simulink model "Punto_3"  (R2020a)
settings: Solver=VariableStepAuto  StartTime=0.0  StopTime=10.0  RelTol=1e-3
undefined symbols (not defined in the file): t0
libraries: simulink x3
settings Model: Creator=nicoquintero  LastModifiedBy=nicoquintero

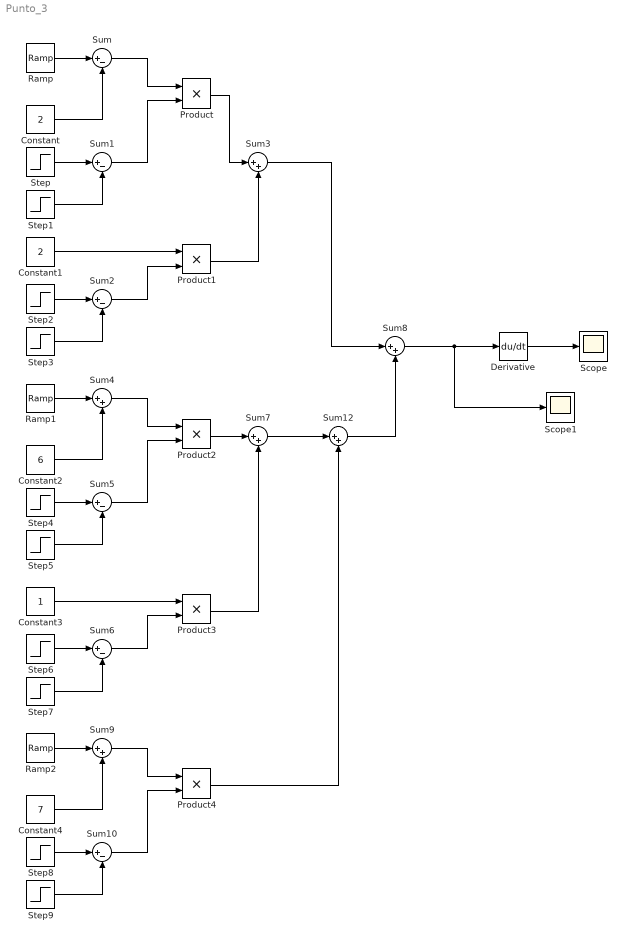
== system Punto_3 ==
  Constant : Constant  Value=2
  Constant1 : Constant  Value=2
  Constant2 : Constant  Value=6
  Constant3 : Constant
  Constant4 : Constant  Value=7
  Derivative : Derivative
  Product{,1..4} (5 alike) : Product
  Ramp : simulink/Sources/Ramp  slope=2  start=t0  InitialOutput=0
  Ramp1 : simulink/Sources/Ramp  slope=-1  start=t0  InitialOutput=0
  Ramp2 : simulink/Sources/Ramp  slope=-1  start=t0  InitialOutput=0
  Scope : Scope
  Scope1 : Scope
  Step : Step  Time=t0  SampleTime=0
  Step1 : Step  Time=t0+2  SampleTime=0
  Step2 : Step  Time=t0+2  SampleTime=0
  Step3 : Step  Time=t0+3  SampleTime=0
  Step4 : Step  Time=t0+3  SampleTime=0
  Step5 : Step  Time=t0+5  SampleTime=0
  Step6 : Step  Time=t0+5  SampleTime=0
  Step7 : Step  Time=t0+6  SampleTime=0
  Step8 : Step  Time=t0+6  SampleTime=0
  Step9 : Step  Time=t0+8  SampleTime=0
  Sum{,1..2,5..6,10} (6 alike) : Sum  Inputs=|+-
  Sum{3..4,7..9,12} (6 alike) : Sum  Inputs=|++
  wires:
  Ramp/1 -> Sum/1
  Constant/1 -> Sum/2
  Step/1 -> Sum1/1
  Step1/1 -> Sum1/2
  Sum1/1 -> Product/2
  Sum/1 -> Product/1
  Step2/1 -> Sum2/1
  Step3/1 -> Sum2/2
  Constant1/1 -> Product1/1
  Sum2/1 -> Product1/2
  Product1/1 -> Sum3/2
  Product/1 -> Sum3/1
  Step5/1 -> Sum5/2
  Sum5/1 -> Product2/2
  Step4/1 -> Sum5/1
  Constant2/1 -> Sum4/2
  Sum4/1 -> Product2/1
  Ramp1/1 -> Sum4/1
  Step7/1 -> Sum6/2
  Constant3/1 -> Product3/1
  Product3/1 -> Sum7/2
  Sum6/1 -> Product3/2
  Step6/1 -> Sum6/1
  Product2/1 -> Sum7/1
  Sum3/1 -> Sum8/1
  Constant4/1 -> Sum9/2
  Step9/1 -> Sum10/2
  Step8/1 -> Sum10/1
  Sum10/1 -> Product4/2
  Ramp2/1 -> Sum9/1
  Sum9/1 -> Product4/1
  Sum8/1 -> Scope1/1, Derivative/1
  Derivative/1 -> Scope/1
  Product4/1 -> Sum12/2
  Sum7/1 -> Sum12/1
  Sum12/1 -> Sum8/2
